simulink model "DatcomForceMoment"  (Simulink 8.8)
settings: Solver=FixedStepDiscrete  StartTime=0.0  StopTime=0.1  FixedStep=.1  RelTol=1e-3
values from neighbouring files (symbols this model uses):
  nfs = PlaneData('SI')    [AFDSimInit.m]    (also in AFDSimInitDatcom.m; TransferFunction.m = PlaneData('Imperial'))
undefined symbols (not defined in the file or in its folder): datcom, Newton, Raphson, sigbuilder_block
libraries: aerolibutil x12, aerolibtransform2 x1, aerolibasang x1
(part 2 of 2)

== system DatcomForceMoment/Digital DATCOM v1.0.2/Dynamic Contribution/Aerodynamic Forces and Moments Stability Axis/Force Transformation ==
  Vb : Inport
  Property-In-Stability (PIS) : Inport  Port=2
  Body2Stability : Subsystem
  "Incidence, Sideslip, & Airspeed" : Subsystem
      mask Display:
      | port_label('input',1,'V_b','texmode','on');
      | port_label('output',1,'\alpha','texmode','on');
      | port_label('output',2,'\beta','texmode','on');
      | port_label('output',3,'V','texmode','on');
  Product : Product  Multiplication=Matrix(*)  RndMeth=Zero
  Terminator : Terminator
  Terminator1 : Terminator
  Transpose : Math  Operator=transpose  SaturateOnIntegerOverflow=on
  Property-In-Body (PIB) : Outport
  wires:
  Product/1 -> Property-In-Body (PIB)/1
  Property-In-Stability (PIS)/1 -> Product/2
  "Incidence, Sideslip, & Airspeed"/1(Alpha) -> Body2Stability/1(alpha)
  Body2Stability/1(Ts/b) -> Transpose/1
  Transpose/1 -> Product/1  "Stability2Body"
  Vb/1 -> "Incidence, Sideslip, & Airspeed"/1(Vb)
  "Incidence, Sideslip, & Airspeed"/2(Beta) -> Terminator/1
  "Incidence, Sideslip, & Airspeed"/3(V) -> Terminator1/1

== system DatcomForceMoment/Digital DATCOM v1.0.2/Dynamic Contribution/Aerodynamic Forces and Moments Stability Axis/Moment Transformation ==
  Vb : Inport
  Property-In-Stability (PIS) : Inport  Port=2
  Body2Stability : Subsystem
  "Incidence, Sideslip, & Airspeed" : Subsystem
      mask Display:
      | port_label('input',1,'V_b','texmode','on');
      | port_label('output',1,'\alpha','texmode','on');
      | port_label('output',2,'\beta','texmode','on');
      | port_label('output',3,'V','texmode','on');
  Product : Product  Multiplication=Matrix(*)  RndMeth=Zero
  Terminator : Terminator
  Terminator1 : Terminator
  Transpose : Math  Operator=transpose  SaturateOnIntegerOverflow=on
  Property-In-Body (PIB) : Outport
  wires:
  "Incidence, Sideslip, & Airspeed"/3(V) -> Terminator1/1
  "Incidence, Sideslip, & Airspeed"/2(Beta) -> Terminator/1
  Vb/1 -> "Incidence, Sideslip, & Airspeed"/1(Vb)
  Transpose/1 -> Product/1  "Stability2Body"
  Body2Stability/1(Ts/b) -> Transpose/1
  "Incidence, Sideslip, & Airspeed"/1(Alpha) -> Body2Stability/1(alpha)
  Property-In-Stability (PIS)/1 -> Product/2
  Product/1 -> Property-In-Body (PIB)/1

== system DatcomForceMoment/Digital DATCOM v1.0.2/Static Contribution/Aerodynamic Forces and Moments/CG-CP Transformation ==
  Vb : Inport
  Property-In-Stability (PIS) : Inport  Port=2
  Body2Stability : Subsystem
  "Incidence, Sideslip, & Airspeed" : Subsystem
      mask Display:
      | port_label('input',1,'V_b','texmode','on');
      | port_label('output',1,'\alpha','texmode','on');
      | port_label('output',2,'\beta','texmode','on');
      | port_label('output',3,'V','texmode','on');
  Product : Product  Multiplication=Matrix(*)  RndMeth=Zero
  Terminator : Terminator
  Terminator1 : Terminator
  Transpose : Math  Operator=transpose  SaturateOnIntegerOverflow=on
  Property-In-Body (PIB) : Outport
  wires:
  Product/1 -> Property-In-Body (PIB)/1
  Property-In-Stability (PIS)/1 -> Product/2
  "Incidence, Sideslip, & Airspeed"/1(Alpha) -> Body2Stability/1(alpha)
  Body2Stability/1(Ts/b) -> Transpose/1
  Transpose/1 -> Product/1  "Stability2Body"
  Vb/1 -> "Incidence, Sideslip, & Airspeed"/1(Vb)
  "Incidence, Sideslip, & Airspeed"/2(Beta) -> Terminator/1
  "Incidence, Sideslip, & Airspeed"/3(V) -> Terminator1/1

== system DatcomForceMoment/Digital DATCOM v1.0.2/Static Contribution/Aerodynamic Forces and Moments/Force Transformation ==
  Vb : Inport
  Property-In-Stability (PIS) : Inport  Port=2
  Body2Stability : Subsystem
  "Incidence, Sideslip, & Airspeed" : Subsystem
      mask Display:
      | port_label('input',1,'V_b','texmode','on');
      | port_label('output',1,'\alpha','texmode','on');
      | port_label('output',2,'\beta','texmode','on');
      | port_label('output',3,'V','texmode','on');
  Product : Product  Multiplication=Matrix(*)  RndMeth=Zero
  Terminator : Terminator
  Terminator1 : Terminator
  Transpose : Math  Operator=transpose  SaturateOnIntegerOverflow=on
  Property-In-Body (PIB) : Outport
  wires:
  Product/1 -> Property-In-Body (PIB)/1
  Property-In-Stability (PIS)/1 -> Product/2
  "Incidence, Sideslip, & Airspeed"/1(Alpha) -> Body2Stability/1(alpha)
  Body2Stability/1(Ts/b) -> Transpose/1
  Transpose/1 -> Product/1  "Stability2Body"
  Vb/1 -> "Incidence, Sideslip, & Airspeed"/1(Vb)
  "Incidence, Sideslip, & Airspeed"/2(Beta) -> Terminator/1
  "Incidence, Sideslip, & Airspeed"/3(V) -> Terminator1/1

== system DatcomForceMoment/Digital DATCOM v1.0.2/Static Contribution/Aerodynamic Forces and Moments/Moment Transformation ==
  Vb : Inport
  Property-In-Stability (PIS) : Inport  Port=2
  Body2Stability : Subsystem
  "Incidence, Sideslip, & Airspeed" : Subsystem
      mask Display:
      | port_label('input',1,'V_b','texmode','on');
      | port_label('output',1,'\alpha','texmode','on');
      | port_label('output',2,'\beta','texmode','on');
      | port_label('output',3,'V','texmode','on');
  Product : Product  Multiplication=Matrix(*)  RndMeth=Zero
  Terminator : Terminator
  Terminator1 : Terminator
  Transpose : Math  Operator=transpose  SaturateOnIntegerOverflow=on
  Property-In-Body (PIB) : Outport
  wires:
  "Incidence, Sideslip, & Airspeed"/3(V) -> Terminator1/1
  "Incidence, Sideslip, & Airspeed"/2(Beta) -> Terminator/1
  Vb/1 -> "Incidence, Sideslip, & Airspeed"/1(Vb)
  Transpose/1 -> Product/1  "Stability2Body"
  Body2Stability/1(Ts/b) -> Transpose/1
  "Incidence, Sideslip, & Airspeed"/1(Alpha) -> Body2Stability/1(alpha)
  Property-In-Stability (PIS)/1 -> Product/2
  Product/1 -> Property-In-Body (PIB)/1

== system DatcomForceMoment/Digital DATCOM v1.0.2/Deflection/Aerodynamic Forces and Moments/CG-CP Transformation/Body2Stability ==
  alpha : Inport
  Constant{,1,3..4} (4 alike) : Constant  Value=0
  Constant2 : Constant
  Create 3x3 Matrix : aerolibutil/Create 3x3 Matrix
  Trigonometric Function2 : Trigonometry  Operator=sincos
  Unary Minus : UnaryMinus
  Ts/b : Outport
  wires:
  alpha/1 -> Trigonometric Function2/1
  Trigonometric Function2/2 -> Create 3x3 Matrix/9, Create 3x3 Matrix/1
  Constant4/1 -> Create 3x3 Matrix/8
  Unary Minus/1 -> Create 3x3 Matrix/7
  Trigonometric Function2/1 -> Unary Minus/1, Create 3x3 Matrix/3
  Constant3/1 -> Create 3x3 Matrix/6
  Constant2/1 -> Create 3x3 Matrix/5
  Constant1/1 -> Create 3x3 Matrix/4
  Constant/1 -> Create 3x3 Matrix/2
  Create 3x3 Matrix/1 -> Ts/b/1

== system DatcomForceMoment/Digital DATCOM v1.0.2/Deflection/Aerodynamic Forces and Moments/CG-CP Transformation/Incidence, Sideslip, & Airspeed ==
  Vb : Inport  Unit=m/s
  Airspeed : Sqrt  AlgorithmType=Newton-Raphson  SaturateOnIntegerOverflow=on
  Dot Product : DotProduct  InputSameDT=on  OutDataTypeStr=Inherit: Inherit via internal rule
  Incidence : Trigonometry  Operator=atan2
  Product : Product  Inputs=*/  SaturateOnIntegerOverflow=on  OutDataTypeStr=Inherit: Same as first input
  Selector : Selector  InputPortWidth=3  IndexOptions=Index vector (dialog)  Indices=[2]  OutputSizes=1
  Selector1 : Selector  InputPortWidth=3  IndexOptions=Index vector (dialog)  Indices=[3]  OutputSizes=1
  Selector2 : Selector  InputPortWidth=3  IndexOptions=Index vector (dialog)  Indices=[1]  OutputSizes=1
  Sideslip : Trigonometry  Operator=asin
  Alpha : Outport  Unit=rad  InitialOutput=0
  Beta : Outport  Port=2  Unit=rad  InitialOutput=0
  V : Outport  Port=3  Unit=m/s  InitialOutput=0
  wires:
  Selector/1 -> Product/1
  Sideslip/1 -> Beta/1
  Vb/1 -> Dot Product/2, Dot Product/1, Selector/1, Selector2/1, Selector1/1
  Incidence/1 -> Alpha/1
  Airspeed/1 -> V/1, Product/2
  Dot Product/1 -> Airspeed/1
  Selector2/1 -> Incidence/2
  Selector1/1 -> Incidence/1
  Product/1 -> Sideslip/1

== system DatcomForceMoment/Digital DATCOM v1.0.2/Deflection/Aerodynamic Forces and Moments/Force Transformation/Body2Stability ==
  alpha : Inport
  Constant{,1,3..4} (4 alike) : Constant  Value=0
  Constant2 : Constant
  Create 3x3 Matrix : aerolibutil/Create 3x3 Matrix
  Trigonometric Function2 : Trigonometry  Operator=sincos
  Unary Minus : UnaryMinus
  Ts/b : Outport
  wires:
  alpha/1 -> Trigonometric Function2/1
  Trigonometric Function2/2 -> Create 3x3 Matrix/9, Create 3x3 Matrix/1
  Constant4/1 -> Create 3x3 Matrix/8
  Unary Minus/1 -> Create 3x3 Matrix/7
  Trigonometric Function2/1 -> Unary Minus/1, Create 3x3 Matrix/3
  Constant3/1 -> Create 3x3 Matrix/6
  Constant2/1 -> Create 3x3 Matrix/5
  Constant1/1 -> Create 3x3 Matrix/4
  Constant/1 -> Create 3x3 Matrix/2
  Create 3x3 Matrix/1 -> Ts/b/1

== system DatcomForceMoment/Digital DATCOM v1.0.2/Deflection/Aerodynamic Forces and Moments/Force Transformation/Incidence, Sideslip, & Airspeed ==
  Vb : Inport  Unit=m/s
  Airspeed : Sqrt  AlgorithmType=Newton-Raphson  SaturateOnIntegerOverflow=on
  Dot Product : DotProduct  InputSameDT=on  OutDataTypeStr=Inherit: Inherit via internal rule
  Incidence : Trigonometry  Operator=atan2
  Product : Product  Inputs=*/  SaturateOnIntegerOverflow=on  OutDataTypeStr=Inherit: Same as first input
  Selector : Selector  InputPortWidth=3  IndexOptions=Index vector (dialog)  Indices=[2]  OutputSizes=1
  Selector1 : Selector  InputPortWidth=3  IndexOptions=Index vector (dialog)  Indices=[3]  OutputSizes=1
  Selector2 : Selector  InputPortWidth=3  IndexOptions=Index vector (dialog)  Indices=[1]  OutputSizes=1
  Sideslip : Trigonometry  Operator=asin
  Alpha : Outport  Unit=rad  InitialOutput=0
  Beta : Outport  Port=2  Unit=rad  InitialOutput=0
  V : Outport  Port=3  Unit=m/s  InitialOutput=0
  wires:
  Selector/1 -> Product/1
  Sideslip/1 -> Beta/1
  Vb/1 -> Dot Product/2, Dot Product/1, Selector/1, Selector2/1, Selector1/1
  Incidence/1 -> Alpha/1
  Airspeed/1 -> V/1, Product/2
  Dot Product/1 -> Airspeed/1
  Selector2/1 -> Incidence/2
  Selector1/1 -> Incidence/1
  Product/1 -> Sideslip/1

== system DatcomForceMoment/Digital DATCOM v1.0.2/Deflection/Aerodynamic Forces and Moments/Moment Transformation/Body2Stability ==
  alpha : Inport
  Constant{,1,3..4} (4 alike) : Constant  Value=0
  Constant2 : Constant
  Create 3x3 Matrix : aerolibutil/Create 3x3 Matrix
  Trigonometric Function2 : Trigonometry  Operator=sincos
  Unary Minus : UnaryMinus
  Ts/b : Outport
  wires:
  Create 3x3 Matrix/1 -> Ts/b/1
  Constant/1 -> Create 3x3 Matrix/2
  Constant1/1 -> Create 3x3 Matrix/4
  Constant2/1 -> Create 3x3 Matrix/5
  Constant3/1 -> Create 3x3 Matrix/6
  Trigonometric Function2/1 -> Create 3x3 Matrix/3, Unary Minus/1
  Unary Minus/1 -> Create 3x3 Matrix/7
  Constant4/1 -> Create 3x3 Matrix/8
  Trigonometric Function2/2 -> Create 3x3 Matrix/1, Create 3x3 Matrix/9
  alpha/1 -> Trigonometric Function2/1

== system DatcomForceMoment/Digital DATCOM v1.0.2/Deflection/Aerodynamic Forces and Moments/Moment Transformation/Incidence, Sideslip, & Airspeed ==
  Vb : Inport  Unit=m/s
  Airspeed : Sqrt  AlgorithmType=Newton-Raphson  SaturateOnIntegerOverflow=on
  Dot Product : DotProduct  InputSameDT=on  OutDataTypeStr=Inherit: Inherit via internal rule
  Incidence : Trigonometry  Operator=atan2
  Product : Product  Inputs=*/  SaturateOnIntegerOverflow=on  OutDataTypeStr=Inherit: Same as first input
  Selector : Selector  InputPortWidth=3  IndexOptions=Index vector (dialog)  Indices=[2]  OutputSizes=1
  Selector1 : Selector  InputPortWidth=3  IndexOptions=Index vector (dialog)  Indices=[3]  OutputSizes=1
  Selector2 : Selector  InputPortWidth=3  IndexOptions=Index vector (dialog)  Indices=[1]  OutputSizes=1
  Sideslip : Trigonometry  Operator=asin
  Alpha : Outport  Unit=rad  InitialOutput=0
  Beta : Outport  Port=2  Unit=rad  InitialOutput=0
  V : Outport  Port=3  Unit=m/s  InitialOutput=0
  wires:
  Product/1 -> Sideslip/1
  Selector1/1 -> Incidence/1
  Selector2/1 -> Incidence/2
  Dot Product/1 -> Airspeed/1
  Airspeed/1 -> Product/2, V/1
  Incidence/1 -> Alpha/1
  Vb/1 -> Selector1/1, Selector2/1, Selector/1, Dot Product/1, Dot Product/2
  Sideslip/1 -> Beta/1
  Selector/1 -> Product/1

== system DatcomForceMoment/Digital DATCOM v1.0.2/Dynamic Contribution/Aerodynamic Forces and Moments Stability Axis/CG-CP Transformation/Body2Stability ==
  alpha : Inport
  Constant{,1,3..4} (4 alike) : Constant  Value=0
  Constant2 : Constant
  Create 3x3 Matrix : aerolibutil/Create 3x3 Matrix
  Trigonometric Function2 : Trigonometry  Operator=sincos
  Unary Minus : UnaryMinus
  Ts/b : Outport
  wires:
  alpha/1 -> Trigonometric Function2/1
  Trigonometric Function2/2 -> Create 3x3 Matrix/9, Create 3x3 Matrix/1
  Constant4/1 -> Create 3x3 Matrix/8
  Unary Minus/1 -> Create 3x3 Matrix/7
  Trigonometric Function2/1 -> Unary Minus/1, Create 3x3 Matrix/3
  Constant3/1 -> Create 3x3 Matrix/6
  Constant2/1 -> Create 3x3 Matrix/5
  Constant1/1 -> Create 3x3 Matrix/4
  Constant/1 -> Create 3x3 Matrix/2
  Create 3x3 Matrix/1 -> Ts/b/1

== system DatcomForceMoment/Digital DATCOM v1.0.2/Dynamic Contribution/Aerodynamic Forces and Moments Stability Axis/CG-CP Transformation/Incidence, Sideslip, & Airspeed ==
  Vb : Inport  Unit=m/s
  Airspeed : Sqrt  AlgorithmType=Newton-Raphson  SaturateOnIntegerOverflow=on
  Dot Product : DotProduct  InputSameDT=on  OutDataTypeStr=Inherit: Inherit via internal rule
  Incidence : Trigonometry  Operator=atan2
  Product : Product  Inputs=*/  SaturateOnIntegerOverflow=on  OutDataTypeStr=Inherit: Same as first input
  Selector : Selector  InputPortWidth=3  IndexOptions=Index vector (dialog)  Indices=[2]  OutputSizes=1
  Selector1 : Selector  InputPortWidth=3  IndexOptions=Index vector (dialog)  Indices=[3]  OutputSizes=1
  Selector2 : Selector  InputPortWidth=3  IndexOptions=Index vector (dialog)  Indices=[1]  OutputSizes=1
  Sideslip : Trigonometry  Operator=asin
  Alpha : Outport  Unit=rad  InitialOutput=0
  Beta : Outport  Port=2  Unit=rad  InitialOutput=0
  V : Outport  Port=3  Unit=m/s  InitialOutput=0
  wires:
  Selector/1 -> Product/1
  Sideslip/1 -> Beta/1
  Vb/1 -> Dot Product/2, Dot Product/1, Selector/1, Selector2/1, Selector1/1
  Incidence/1 -> Alpha/1
  Airspeed/1 -> V/1, Product/2
  Dot Product/1 -> Airspeed/1
  Selector2/1 -> Incidence/2
  Selector1/1 -> Incidence/1
  Product/1 -> Sideslip/1

== system DatcomForceMoment/Digital DATCOM v1.0.2/Dynamic Contribution/Aerodynamic Forces and Moments Stability Axis/Force Transformation/Body2Stability ==
  alpha : Inport
  Constant{,1,3..4} (4 alike) : Constant  Value=0
  Constant2 : Constant
  Create 3x3 Matrix : aerolibutil/Create 3x3 Matrix
  Trigonometric Function2 : Trigonometry  Operator=sincos
  Unary Minus : UnaryMinus
  Ts/b : Outport
  wires:
  alpha/1 -> Trigonometric Function2/1
  Trigonometric Function2/2 -> Create 3x3 Matrix/9, Create 3x3 Matrix/1
  Constant4/1 -> Create 3x3 Matrix/8
  Unary Minus/1 -> Create 3x3 Matrix/7
  Trigonometric Function2/1 -> Unary Minus/1, Create 3x3 Matrix/3
  Constant3/1 -> Create 3x3 Matrix/6
  Constant2/1 -> Create 3x3 Matrix/5
  Constant1/1 -> Create 3x3 Matrix/4
  Constant/1 -> Create 3x3 Matrix/2
  Create 3x3 Matrix/1 -> Ts/b/1

== system DatcomForceMoment/Digital DATCOM v1.0.2/Dynamic Contribution/Aerodynamic Forces and Moments Stability Axis/Force Transformation/Incidence, Sideslip, & Airspeed ==
  Vb : Inport  Unit=m/s
  Airspeed : Sqrt  AlgorithmType=Newton-Raphson  SaturateOnIntegerOverflow=on
  Dot Product : DotProduct  InputSameDT=on  OutDataTypeStr=Inherit: Inherit via internal rule
  Incidence : Trigonometry  Operator=atan2
  Product : Product  Inputs=*/  SaturateOnIntegerOverflow=on  OutDataTypeStr=Inherit: Same as first input
  Selector : Selector  InputPortWidth=3  IndexOptions=Index vector (dialog)  Indices=[2]  OutputSizes=1
  Selector1 : Selector  InputPortWidth=3  IndexOptions=Index vector (dialog)  Indices=[3]  OutputSizes=1
  Selector2 : Selector  InputPortWidth=3  IndexOptions=Index vector (dialog)  Indices=[1]  OutputSizes=1
  Sideslip : Trigonometry  Operator=asin
  Alpha : Outport  Unit=rad  InitialOutput=0
  Beta : Outport  Port=2  Unit=rad  InitialOutput=0
  V : Outport  Port=3  Unit=m/s  InitialOutput=0
  wires:
  Selector/1 -> Product/1
  Sideslip/1 -> Beta/1
  Vb/1 -> Dot Product/2, Dot Product/1, Selector/1, Selector2/1, Selector1/1
  Incidence/1 -> Alpha/1
  Airspeed/1 -> V/1, Product/2
  Dot Product/1 -> Airspeed/1
  Selector2/1 -> Incidence/2
  Selector1/1 -> Incidence/1
  Product/1 -> Sideslip/1

== system DatcomForceMoment/Digital DATCOM v1.0.2/Dynamic Contribution/Aerodynamic Forces and Moments Stability Axis/Moment Transformation/Body2Stability ==
  alpha : Inport
  Constant{,1,3..4} (4 alike) : Constant  Value=0
  Constant2 : Constant
  Create 3x3 Matrix : aerolibutil/Create 3x3 Matrix
  Trigonometric Function2 : Trigonometry  Operator=sincos
  Unary Minus : UnaryMinus
  Ts/b : Outport
  wires:
  Create 3x3 Matrix/1 -> Ts/b/1
  Constant/1 -> Create 3x3 Matrix/2
  Constant1/1 -> Create 3x3 Matrix/4
  Constant2/1 -> Create 3x3 Matrix/5
  Constant3/1 -> Create 3x3 Matrix/6
  Trigonometric Function2/1 -> Create 3x3 Matrix/3, Unary Minus/1
  Unary Minus/1 -> Create 3x3 Matrix/7
  Constant4/1 -> Create 3x3 Matrix/8
  Trigonometric Function2/2 -> Create 3x3 Matrix/1, Create 3x3 Matrix/9
  alpha/1 -> Trigonometric Function2/1

== system DatcomForceMoment/Digital DATCOM v1.0.2/Dynamic Contribution/Aerodynamic Forces and Moments Stability Axis/Moment Transformation/Incidence, Sideslip, & Airspeed ==
  Vb : Inport  Unit=m/s
  Airspeed : Sqrt  AlgorithmType=Newton-Raphson  SaturateOnIntegerOverflow=on
  Dot Product : DotProduct  InputSameDT=on  OutDataTypeStr=Inherit: Inherit via internal rule
  Incidence : Trigonometry  Operator=atan2
  Product : Product  Inputs=*/  SaturateOnIntegerOverflow=on  OutDataTypeStr=Inherit: Same as first input
  Selector : Selector  InputPortWidth=3  IndexOptions=Index vector (dialog)  Indices=[2]  OutputSizes=1
  Selector1 : Selector  InputPortWidth=3  IndexOptions=Index vector (dialog)  Indices=[3]  OutputSizes=1
  Selector2 : Selector  InputPortWidth=3  IndexOptions=Index vector (dialog)  Indices=[1]  OutputSizes=1
  Sideslip : Trigonometry  Operator=asin
  Alpha : Outport  Unit=rad  InitialOutput=0
  Beta : Outport  Port=2  Unit=rad  InitialOutput=0
  V : Outport  Port=3  Unit=m/s  InitialOutput=0
  wires:
  Product/1 -> Sideslip/1
  Selector1/1 -> Incidence/1
  Selector2/1 -> Incidence/2
  Dot Product/1 -> Airspeed/1
  Airspeed/1 -> Product/2, V/1
  Incidence/1 -> Alpha/1
  Vb/1 -> Selector1/1, Selector2/1, Selector/1, Dot Product/1, Dot Product/2
  Sideslip/1 -> Beta/1
  Selector/1 -> Product/1

== system DatcomForceMoment/Digital DATCOM v1.0.2/Static Contribution/Aerodynamic Forces and Moments/CG-CP Transformation/Body2Stability ==
  alpha : Inport
  Constant{,1,3..4} (4 alike) : Constant  Value=0
  Constant2 : Constant
  Create 3x3 Matrix : aerolibutil/Create 3x3 Matrix
  Trigonometric Function2 : Trigonometry  Operator=sincos
  Unary Minus : UnaryMinus
  Ts/b : Outport
  wires:
  alpha/1 -> Trigonometric Function2/1
  Trigonometric Function2/2 -> Create 3x3 Matrix/9, Create 3x3 Matrix/1
  Constant4/1 -> Create 3x3 Matrix/8
  Unary Minus/1 -> Create 3x3 Matrix/7
  Trigonometric Function2/1 -> Unary Minus/1, Create 3x3 Matrix/3
  Constant3/1 -> Create 3x3 Matrix/6
  Constant2/1 -> Create 3x3 Matrix/5
  Constant1/1 -> Create 3x3 Matrix/4
  Constant/1 -> Create 3x3 Matrix/2
  Create 3x3 Matrix/1 -> Ts/b/1

== system DatcomForceMoment/Digital DATCOM v1.0.2/Static Contribution/Aerodynamic Forces and Moments/CG-CP Transformation/Incidence, Sideslip, & Airspeed ==
  Vb : Inport  Unit=m/s
  Airspeed : Sqrt  AlgorithmType=Newton-Raphson  SaturateOnIntegerOverflow=on
  Dot Product : DotProduct  InputSameDT=on  OutDataTypeStr=Inherit: Inherit via internal rule
  Incidence : Trigonometry  Operator=atan2
  Product : Product  Inputs=*/  SaturateOnIntegerOverflow=on  OutDataTypeStr=Inherit: Same as first input
  Selector : Selector  InputPortWidth=3  IndexOptions=Index vector (dialog)  Indices=[2]  OutputSizes=1
  Selector1 : Selector  InputPortWidth=3  IndexOptions=Index vector (dialog)  Indices=[3]  OutputSizes=1
  Selector2 : Selector  InputPortWidth=3  IndexOptions=Index vector (dialog)  Indices=[1]  OutputSizes=1
  Sideslip : Trigonometry  Operator=asin
  Alpha : Outport  Unit=rad  InitialOutput=0
  Beta : Outport  Port=2  Unit=rad  InitialOutput=0
  V : Outport  Port=3  Unit=m/s  InitialOutput=0
  wires:
  Selector/1 -> Product/1
  Sideslip/1 -> Beta/1
  Vb/1 -> Dot Product/2, Dot Product/1, Selector/1, Selector2/1, Selector1/1
  Incidence/1 -> Alpha/1
  Airspeed/1 -> V/1, Product/2
  Dot Product/1 -> Airspeed/1
  Selector2/1 -> Incidence/2
  Selector1/1 -> Incidence/1
  Product/1 -> Sideslip/1

== system DatcomForceMoment/Digital DATCOM v1.0.2/Static Contribution/Aerodynamic Forces and Moments/Force Transformation/Body2Stability ==
  alpha : Inport
  Constant{,1,3..4} (4 alike) : Constant  Value=0
  Constant2 : Constant
  Create 3x3 Matrix : aerolibutil/Create 3x3 Matrix
  Trigonometric Function2 : Trigonometry  Operator=sincos
  Unary Minus : UnaryMinus
  Ts/b : Outport
  wires:
  alpha/1 -> Trigonometric Function2/1
  Trigonometric Function2/2 -> Create 3x3 Matrix/9, Create 3x3 Matrix/1
  Constant4/1 -> Create 3x3 Matrix/8
  Unary Minus/1 -> Create 3x3 Matrix/7
  Trigonometric Function2/1 -> Unary Minus/1, Create 3x3 Matrix/3
  Constant3/1 -> Create 3x3 Matrix/6
  Constant2/1 -> Create 3x3 Matrix/5
  Constant1/1 -> Create 3x3 Matrix/4
  Constant/1 -> Create 3x3 Matrix/2
  Create 3x3 Matrix/1 -> Ts/b/1

== system DatcomForceMoment/Digital DATCOM v1.0.2/Static Contribution/Aerodynamic Forces and Moments/Force Transformation/Incidence, Sideslip, & Airspeed ==
  Vb : Inport  Unit=m/s
  Airspeed : Sqrt  AlgorithmType=Newton-Raphson  SaturateOnIntegerOverflow=on
  Dot Product : DotProduct  InputSameDT=on  OutDataTypeStr=Inherit: Inherit via internal rule
  Incidence : Trigonometry  Operator=atan2
  Product : Product  Inputs=*/  SaturateOnIntegerOverflow=on  OutDataTypeStr=Inherit: Same as first input
  Selector : Selector  InputPortWidth=3  IndexOptions=Index vector (dialog)  Indices=[2]  OutputSizes=1
  Selector1 : Selector  InputPortWidth=3  IndexOptions=Index vector (dialog)  Indices=[3]  OutputSizes=1
  Selector2 : Selector  InputPortWidth=3  IndexOptions=Index vector (dialog)  Indices=[1]  OutputSizes=1
  Sideslip : Trigonometry  Operator=asin
  Alpha : Outport  Unit=rad  InitialOutput=0
  Beta : Outport  Port=2  Unit=rad  InitialOutput=0
  V : Outport  Port=3  Unit=m/s  InitialOutput=0
  wires:
  Selector/1 -> Product/1
  Sideslip/1 -> Beta/1
  Vb/1 -> Dot Product/2, Dot Product/1, Selector/1, Selector2/1, Selector1/1
  Incidence/1 -> Alpha/1
  Airspeed/1 -> V/1, Product/2
  Dot Product/1 -> Airspeed/1
  Selector2/1 -> Incidence/2
  Selector1/1 -> Incidence/1
  Product/1 -> Sideslip/1

== system DatcomForceMoment/Digital DATCOM v1.0.2/Static Contribution/Aerodynamic Forces and Moments/Moment Transformation/Body2Stability ==
  alpha : Inport
  Constant{,1,3..4} (4 alike) : Constant  Value=0
  Constant2 : Constant
  Create 3x3 Matrix : aerolibutil/Create 3x3 Matrix
  Trigonometric Function2 : Trigonometry  Operator=sincos
  Unary Minus : UnaryMinus
  Ts/b : Outport
  wires:
  Create 3x3 Matrix/1 -> Ts/b/1
  Constant/1 -> Create 3x3 Matrix/2
  Constant1/1 -> Create 3x3 Matrix/4
  Constant2/1 -> Create 3x3 Matrix/5
  Constant3/1 -> Create 3x3 Matrix/6
  Trigonometric Function2/1 -> Create 3x3 Matrix/3, Unary Minus/1
  Unary Minus/1 -> Create 3x3 Matrix/7
  Constant4/1 -> Create 3x3 Matrix/8
  Trigonometric Function2/2 -> Create 3x3 Matrix/1, Create 3x3 Matrix/9
  alpha/1 -> Trigonometric Function2/1

== system DatcomForceMoment/Digital DATCOM v1.0.2/Static Contribution/Aerodynamic Forces and Moments/Moment Transformation/Incidence, Sideslip, & Airspeed ==
  Vb : Inport  Unit=m/s
  Airspeed : Sqrt  AlgorithmType=Newton-Raphson  SaturateOnIntegerOverflow=on
  Dot Product : DotProduct  InputSameDT=on  OutDataTypeStr=Inherit: Inherit via internal rule
  Incidence : Trigonometry  Operator=atan2
  Product : Product  Inputs=*/  SaturateOnIntegerOverflow=on  OutDataTypeStr=Inherit: Same as first input
  Selector : Selector  InputPortWidth=3  IndexOptions=Index vector (dialog)  Indices=[2]  OutputSizes=1
  Selector1 : Selector  InputPortWidth=3  IndexOptions=Index vector (dialog)  Indices=[3]  OutputSizes=1
  Selector2 : Selector  InputPortWidth=3  IndexOptions=Index vector (dialog)  Indices=[1]  OutputSizes=1
  Sideslip : Trigonometry  Operator=asin
  Alpha : Outport  Unit=rad  InitialOutput=0
  Beta : Outport  Port=2  Unit=rad  InitialOutput=0
  V : Outport  Port=3  Unit=m/s  InitialOutput=0
  wires:
  Product/1 -> Sideslip/1
  Selector1/1 -> Incidence/1
  Selector2/1 -> Incidence/2
  Dot Product/1 -> Airspeed/1
  Airspeed/1 -> Product/2, V/1
  Incidence/1 -> Alpha/1
  Vb/1 -> Selector1/1, Selector2/1, Selector/1, Dot Product/1, Dot Product/2
  Sideslip/1 -> Beta/1
  Selector/1 -> Product/1
